simulink model "sl_regulator"  (R2022b)
settings: Solver=ode23t  StartTime=0.0  StopTime=99.7  FixedStep=0.01  MaxStep=0.05  RelTol=1e-3  EnableMultiTasking=on
PreLoadFcn:
  | mdl_puma560
undefined symbols (not defined in the file): hp6, sl_Kd, sl_Kp, slcoulomb
libraries: roblocks x4
settings Model: Creator=pic  LastModifiedBy=sam
settings SolverCC: ZeroCrossControl=DisableAll  AlgebraicLoopSolver=TrustRegion
settings DataIOCC: SaveFormat=Array  SignalLoggingSaveFormat=ModelDataLogs  TimeSaveName=t  OutputSaveName=y  ReturnWorkspaceOutputsName=ctorque
settings OptimizationCC: BlockReduction=off  BooleanDataType=off  ExpressionDepthLimit=2147483647  InitFltsAndDblsToZero=on  LifeSpan=inf
settings DebuggingCC: SaveWithParameterizedLinksMsg=none  UnderspecifiedInitializationDetection=Classic  MergeDetectMultiDrivingBlocksExec=none  SignalResolutionControl=TryResolveAllWithWarning  MultiTaskDSMMsg=warning  MultiTaskCondExecSysMsg=none  FcnCallInpInsideContextMsg=warning  UnconnectedInputMsg=warning  UnconnectedOutputMsg=warning  UnconnectedLineMsg=warning  AllowSymbolicDim=off  StateNameClashWarn=warning  SFUnexpectedBacktrackingDiag=warning  SFNoUnconditionalDefaultTransitionDiag=warning  SFExecutionAtInitializationDiag=none  SFMachineParentedDataDiag=warning  ArithmeticOperatorsInVariantConditions=warning
settings HardwareCC: ProdBitPerPointer=32  ProdBitPerSizeT=32  ProdBitPerPtrDiffT=32  ProdLargestAtomicFloat=None  ProdIntDivRoundTo=Undefined  ProdEndianess=Unspecified  ProdWordSize=32  ProdHWDeviceType=32-bit Generic  TargetUnknown=on
settings ModelReferenceCC: EnableRefExpFcnMdlSchedulingChecks=on  PropagateSignalLabelsOutOfModel=off
settings SFSimCC: SimUseLocalCustomCode=off  CustomCodeUndefinedFunction=UseInterfaceOnly
settings RTWCC: RTWUseLocalCustomCode=off
settings CodeAppCC: StateflowObjectComments=on
settings GRTTargetCC: TargetLangStandard=C89/C90 (ANSI)  ModelReferenceCompliant=off  CompOptLevelCompliant=off  CombineOutputUpdateFcns=off  MatFileLogging=off  GRTInterface=on
settings ConfigComp: CovMetricSettings=dw  CovSaveCumulativeToWorkspaceVar=on  CovSaveSingleToWorkspaceVar=on  CovExternalEMLEnable=off

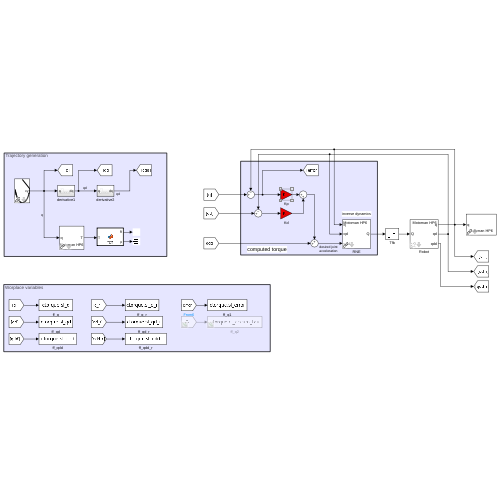
[thumbnail: Simulink's stored preview of the top-level diagram]
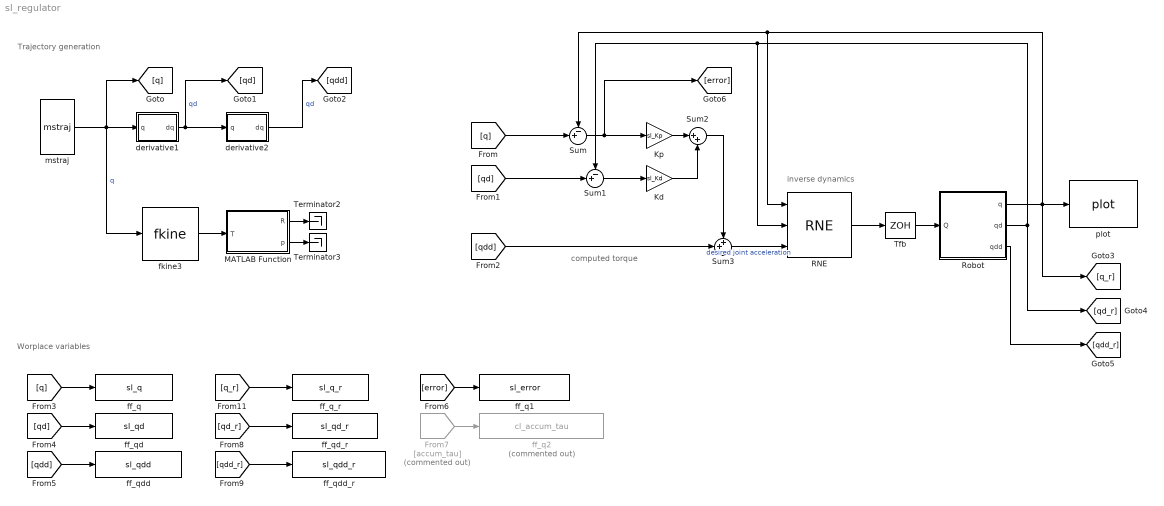
== system sl_regulator ==
  note: inverse dynamics
  note: computed torque
  note: Trajectory generation
  note: Worplace variables
  From7 : From  Commented=on  GotoTag=accum_tau
  Kd : Gain  Gain=sl_Kd  SaturateOnIntegerOverflow=on  OutDataTypeStr=Inherit: Same as input  ParamDataTypeStr=Inherit: Same as input
  Kp : Gain  Gain=sl_Kp  SaturateOnIntegerOverflow=on  OutDataTypeStr=Inherit: Same as input  ParamDataTypeStr=Inherit: Same as input
  MATLAB Function : MATLAB Function  TreatAsAtomicUnit=on
  RNE : roblocks/Arm/RNE  robot=hp6  grav=[0 0 9.81]
  Robot : Subsystem  AncestorBlock=roblocks/Arm/Robot  mask{robot=hp6, q0=[0 0 0 0 0 0]}
      mask prompts: robot "Robot object"; q0 "Initial state"
      mask help: Rigid-body dynamic model of robot.
      mask init:
      | if isa(robot, 'SerialLink')
      |     rname = robot.name;
      |     %fprintf('**robot name is %s\n', rname);
      | else
      |     rname = '';
      |     n = 0
      | end
      settings: LibrarySourceBlock=roblocks/Arm/Robot
      mask Help:
      | Simulates the forward (direct) rigid-body dynamics of the robot described
      | by the given robot object.  For given applied joint torque/force it computes
      | the instaneous joint coordinates, velocities and acclerations.
      | 
      | 
      | <b>Parameters::</b>
      | 
      | robot (SerialLink) a dynamic model of an N-link serial link manipulator
      | q0 (1xN)  Initial joint coordinates
      | 
      | <b>Inputs::</b>
      | 
      | Q (1xN) the generalized joint force (torque or force) required to achieve
      | the motion state (q, qd, qdd).
      | 
      | <b>Outputs::</b>
      | 
      | q (1xN) joint coordinates
      | qd (1xN) joint coordinate velocity
      | qdd (1xN) joint coordinate acceleration
      | 
      | 
      | <b>Notes::</b>
      | 
      | - Required to simulate robot rigid body motion.
      | - Implemented using the recursive Newton-Euler scheme (RNE).
      | - A wrapper for the Toolbox method accel() which in turn depends on the
      |   method rne().
      mask Display:
      | port_label('input', 1, 'Q')
      | port_label('output', 1, 'q')
      | port_label('output', 2, 'qd')
      | port_label('output', 3, 'qdd')
      | text(0.1, 0.9,  rname, 'horizontalAlignment', 'left')
  Sum : Sum  Inputs=-+|  InputSameDT=on  SaturateOnIntegerOverflow=on  OutDataTypeStr=Inherit: Same as first input
  Sum1 : Sum  Inputs=-+|  InputSameDT=on  SaturateOnIntegerOverflow=on  OutDataTypeStr=Inherit: Same as first input
  Sum2 : Sum  Inputs=|++  InputSameDT=on  SaturateOnIntegerOverflow=on  OutDataTypeStr=Inherit: Same as first input
  Sum3 : Sum  Inputs=++|  InputSameDT=on  SaturateOnIntegerOverflow=on  OutDataTypeStr=Inherit: Same as first input
  Terminator2 : Terminator
  Terminator3 : Terminator
  Tfb : ZeroOrderHold  SampleTime=0.005
  derivative1 : Subsystem
  derivative2 : Subsystem
  ff_q : ToWorkspace  VariableName=sl_q  SaveFormat=Structure With Time  SampleTime=-1
  ff_q1 : ToWorkspace  VariableName=sl_error  SaveFormat=Structure With Time  SampleTime=-1
  ff_q2 : ToWorkspace  Commented=on  VariableName=cl_accum_tau  SaveFormat=Structure With Time  SampleTime=-1
  ff_q_r : ToWorkspace  VariableName=sl_q_r  SaveFormat=Structure With Time  SampleTime=-1
  ff_qd : ToWorkspace  VariableName=sl_qd  SaveFormat=Structure With Time  SampleTime=-1
  ff_qd_r : ToWorkspace  VariableName=sl_qd_r  SaveFormat=Structure With Time  SampleTime=-1
  ff_qdd : ToWorkspace  VariableName=sl_qdd  SaveFormat=Structure With Time  SampleTime=-1
  ff_qdd_r : ToWorkspace  VariableName=sl_qdd_r  SaveFormat=Structure With Time  SampleTime=-1
  fkine3 : roblocks/Arm/fkine  robot=hp6
  mstraj : roblocks/Toolbox/mstraj  path=pathFull2  vaxis=[2 2 2 2 2 2]  tseg=[]  dt=0.1  tacc=0.3  setsimtime=on
  plot : roblocks/Arm/plot  robot=hp6  fps=10  holdplot=on
  wires:
  Sum/1 -> [error], Kp/1
  Kp/1 -> Sum2/1
  Robot/1(q) -> [q_r], RNE/1, Sum/1, plot/1
  RNE/1 -> Tfb/1
  [q] -> Sum/2
  [qd] -> Sum1/2
  Sum1/1 -> Kd/1
  Kd/1 -> Sum2/2
  Robot/3(qdd) -> [qdd_r]
  Sum3/1 -> RNE/3  "desired joint acceleration"
  Tfb/1 -> Robot/1(Q)
  Robot/2(qd) -> [qd_r], RNE/2, Sum1/1
  [qdd] -> Sum3/2
  Sum2/1 -> Sum3/1
  derivative1/1(dq) -> derivative2/1(q), [qd]  "qd"
  mstraj/1 -> derivative1/1(q), fkine3/1, [q]  "q"
  MATLAB Function/2(p) -> Terminator3/1
  derivative2/1(dq) -> [qdd]  "qd"
  MATLAB Function/1(R) -> Terminator2/1
  fkine3/1 -> MATLAB Function/1(T)
  [q] -> ff_q/1
  [qd] -> ff_qd/1
  [qdd] -> ff_qdd/1
  [q_r] -> ff_q_r/1
  [error] -> ff_q1/1
  From7/1 -> ff_q2/1
  [qd_r] -> ff_qd_r/1
  [qdd_r] -> ff_qdd_r/1

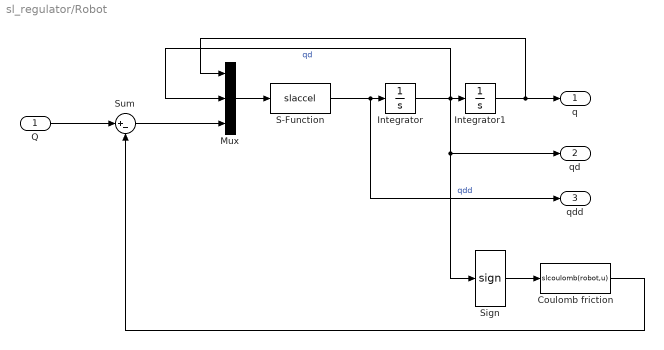
== system sl_regulator/Robot ==
  Q : Inport
  Coulomb friction : MATLABFcn  MATLABFcn=slcoulomb(robot,u)  OutputDimensions=[robot.n 1]  Output1D=off
  Integrator : Integrator
  Integrator1 : Integrator  InitialCondition=q0
  Mux : Mux  Inputs=3
  S-Function : S-Function  FunctionName=slaccel  Parameters=robot  SFunctionDeploymentMode=off  EnableBusSupport=off
  Sign : Signum
  Sum : Sum  Inputs=|+-
  q : Outport  VectorParamsAs1DForOutWhenUnconnected=off
  qd : Outport  Port=2  VectorParamsAs1DForOutWhenUnconnected=off
  qdd : Outport  Port=3  VectorParamsAs1DForOutWhenUnconnected=off
  wires:
  S-Function/1 -> qdd/1, Integrator/1  "qdd"
  Mux/1 -> S-Function/1
  Integrator/1 -> Sign/1, qd/1, Integrator1/1, Mux/2  "qd"
  Integrator1/1 -> q/1, Mux/1
  Q/1 -> Sum/1
  Sum/1 -> Mux/3
  Coulomb friction/1 -> Sum/2
  Sign/1 -> Coulomb friction/1

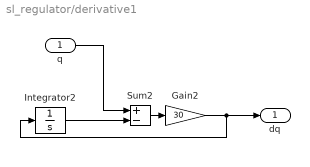
== system sl_regulator/derivative1 ==
  q : Inport
  Gain2 : Gain  Gain=30
  Integrator2 : Integrator
  Sum2 : Sum  Inputs=+-
  dq : Outport
  wires:
  q/1 -> Sum2/1
  Integrator2/1 -> Sum2/2
  Sum2/1 -> Gain2/1
  Gain2/1 -> dq/1, Integrator2/1

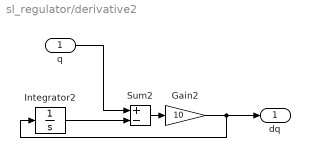
== system sl_regulator/derivative2 ==
  q : Inport
  Gain2 : Gain  Gain=10
  Integrator2 : Integrator
  Sum2 : Sum  Inputs=+-
  dq : Outport
  wires:
  q/1 -> Sum2/1
  Integrator2/1 -> Sum2/2
  Sum2/1 -> Gain2/1
  Gain2/1 -> dq/1, Integrator2/1

== matlab function sl_regulator/MATLAB Function ==
  data: T input; R output; p output
function [R, p] = fcn(T)

p = T([1,2,3],4);
R = T([1,2,3],[1,2,3]);
